simulink model "Tachometer"  (R2016b)
settings: Solver=FixedStepDiscrete  StartTime=0.0  StopTime=10  FixedStep=TimeSteps.ModelStep  RelTol=1e-3
InitFcn:
  | BusInit;
undefined symbols (not defined in the file): DiscIntNeverNeededParam, TimeSteps
settings Model: Creator=KIRTACA  LastModifiedBy=KIRTACA
settings ModelReferenceCC: UpdateModelReferenceTargets=IfOutOfDate  EnableRefExpFcnMdlSchedulingChecks=off  ModelReferenceNumInstancesAllowed=Single  ModelReferenceMinAlgLoopOccurrences=on

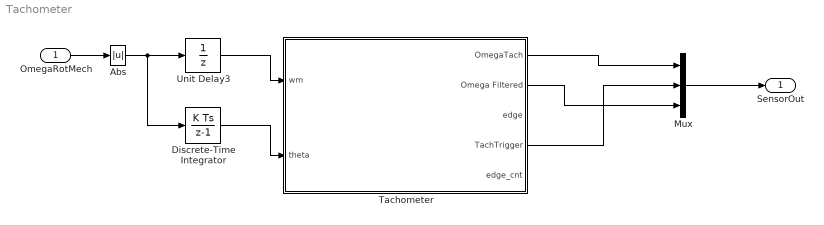
== system Tachometer ==
  OmegaRotMech : Inport  Interpolate=off
  Abs : Abs
  Discrete-Time Integrator : DiscreteIntegrator  InitialConditionSetting=State (most efficient)  SampleTime=-1  ICPrevOutput=DiscIntNeverNeededParam  ICPrevScaledInput=DiscIntNeverNeededParam
  Mux : Mux  Inputs=3
  Tachometer : Subsystem  mask(Tachometer){Clock=1e-6, p=8, tmr_bits=16, Ts=TimeSteps.ModelStep, wmax=4990*2*pi, freq_tmr=1e6, TsSlow=1/500, FirTaps=16}
      mask prompts: FirTaps "Taps"
      mask init:
      | params.Clock     = Clock;
      |         params.p         = p;
      |         params.tmr_bits  = tmr_bits;
      |         params.Ts        = Ts;
      |         params.wmax      = wmax;
      |         params.freq_tmr  = freq_tmr;
      |         params.omega_scl = 0;
      |         params.Speed_max = 0;
      |         params.FirTaps = FirTaps;
  Unit Delay3 : UnitDelay  SampleTime=-1
  SensorOut : Outport
  wires:
  Unit Delay3/1 -> Tachometer/1(wm)
  Discrete-Time Integrator/1 -> Tachometer/2("theta ")
  Abs/1 -> Discrete-Time Integrator/1, Unit Delay3/1
  Mux/1 -> SensorOut/1
  Tachometer/1(OmegaTach) -> Mux/1
  Tachometer/4(TachTrigger) -> Mux/2
  Tachometer/2(Omega Filtered) -> Mux/3
  OmegaRotMech/1 -> Abs/1

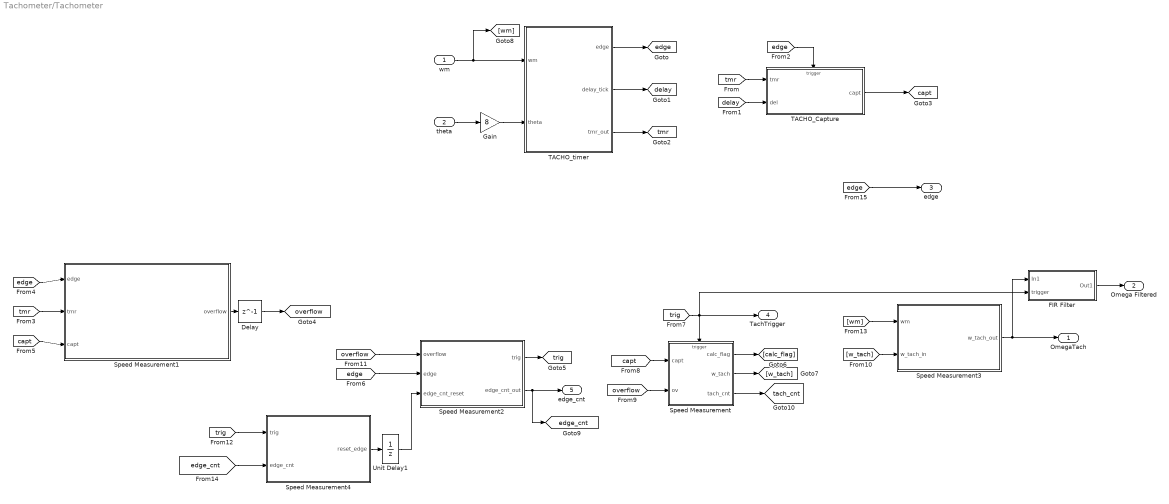
== system Tachometer/Tachometer ==
  wm : Inport
  "theta " : Inport  Port=2
  Delay : Delay  DelayLength=1  InitialCondition=0
  FIR Filter : Subsystem  TreatAsAtomicUnit=on
  Gain : Gain  Gain=8
  Speed Measurement : Subsystem  TreatAsAtomicUnit=on
  Speed Measurement1 : MATLAB Function  TreatAsAtomicUnit=on
  Speed Measurement2 : MATLAB Function  TreatAsAtomicUnit=on
  Speed Measurement3 : MATLAB Function  TreatAsAtomicUnit=on
  Speed Measurement4 : MATLAB Function  TreatAsAtomicUnit=on
  TACHO_Capture : Subsystem  TreatAsAtomicUnit=on
  TACHO_timer : MATLAB Function  TreatAsAtomicUnit=on
  Unit Delay1 : UnitDelay  SampleTime=-1
  OmegaTach : Outport
  Omega Filtered : Outport  Port=2
  edge : Outport  Port=3
  TachTrigger : Outport  Port=4
  edge_cnt : Outport  Port=5
  tag scope: capt=global, delay=global, edge=global, edge_cnt=global, overflow=global, tach_cnt=global, tmr=global, trig=global
  wires:
  Gain/1 -> TACHO_timer/2(theta)
  "theta "/1 -> Gain/1
  [overflow] -> Speed Measurement2/1(overflow)
  wm/1 -> TACHO_timer/1(wm), [wm]
  [overflow] -> Speed Measurement/2(ov)
  [capt] -> Speed Measurement/1(capt)
  [trig] -> TachTrigger/1, FIR Filter/2(trigger), Speed Measurement/Trigger
  Speed Measurement2/1(trig) -> [trig]
  [edge] -> Speed Measurement2/2(edge)
  [capt] -> Speed Measurement1/3(capt)
  [edge] -> Speed Measurement1/1(edge)
  [tmr] -> Speed Measurement1/2(tmr)
  TACHO_Capture/1(capt) -> [capt]
  [edge] -> TACHO_Capture/Trigger
  [tmr] -> TACHO_Capture/1(tmr)
  TACHO_timer/3(tmr_out) -> [tmr]
  TACHO_timer/2(delay_tick) -> [delay]
  TACHO_timer/1(edge) -> [edge]
  Speed Measurement/1(calc_flag) -> [calc_flag]
  Speed Measurement/2(w_tach) -> [w_tach]
  [delay] -> TACHO_Capture/2(del)
  [w_tach] -> Speed Measurement3/2(w_tach_in)
  Speed Measurement3/1(w_tach_out) -> OmegaTach/1, FIR Filter/1(In1)
  [wm] -> Speed Measurement3/1(wm)
  Speed Measurement2/2(edge_cnt_out) -> edge_cnt/1, [edge_cnt]
  Speed Measurement4/1(reset_edge) -> Unit Delay1/1
  [trig] -> Speed Measurement4/1(trig)
  [edge] -> edge/1
  [edge_cnt] -> Speed Measurement4/2(edge_cnt)
  Unit Delay1/1 -> Speed Measurement2/3(edge_cnt_reset)
  Speed Measurement/3(tach_cnt) -> [tach_cnt]
  Speed Measurement1/1(overflow) -> Delay/1
  Delay/1 -> [overflow]
  FIR Filter/1(Out1) -> Omega Filtered/1

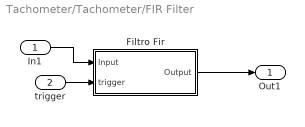
== system Tachometer/Tachometer/FIR Filter ==
  In1 : Inport
  trigger : Inport  Port=2
  Filtro Fir : Subsystem  TreatAsAtomicUnit=on
  Out1 : Outport
  wires:
  In1/1 -> Filtro Fir/1(Input)
  Filtro Fir/1(Output) -> Out1/1
  trigger/1 -> Filtro Fir/2(trigger)

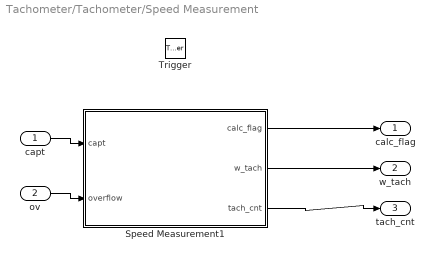
== system Tachometer/Tachometer/Speed Measurement ==
  capt : Inport
  ov : Inport  Port=2
  Trigger : TriggerPort  VariantControl=Variant
  Speed Measurement1 : MATLAB Function  TreatAsAtomicUnit=on
  calc_flag : Outport
  w_tach : Outport  Port=2
  tach_cnt : Outport  Port=3
  wires:
  Speed Measurement1/2(w_tach) -> w_tach/1
  Speed Measurement1/1(calc_flag) -> calc_flag/1
  ov/1 -> Speed Measurement1/2(overflow)
  capt/1 -> Speed Measurement1/1(capt)
  Speed Measurement1/3(tach_cnt) -> tach_cnt/1

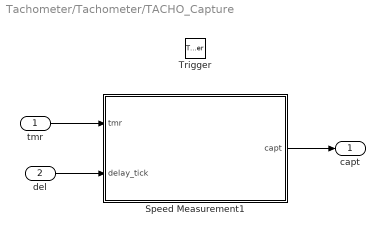
== system Tachometer/Tachometer/TACHO_Capture ==
  tmr : Inport
  del : Inport  Port=2
  Trigger : TriggerPort  VariantControl=Variant
  Speed Measurement1 : MATLAB Function  TreatAsAtomicUnit=on
  capt : Outport
  wires:
  del/1 -> Speed Measurement1/2(delay_tick)
  Speed Measurement1/1(capt) -> capt/1
  tmr/1 -> Speed Measurement1/1(tmr)

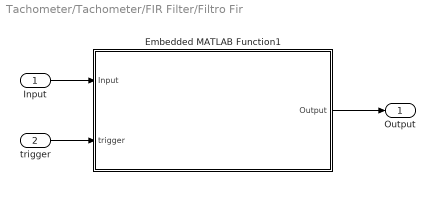
== system Tachometer/Tachometer/FIR Filter/Filtro Fir ==
  Input : Inport
  trigger : Inport  Port=2
  Embedded MATLAB Function1 : MATLAB Function  TreatAsAtomicUnit=on
  Output : Outport
  wires:
  Input/1 -> Embedded MATLAB Function1/1(Input)
  Embedded MATLAB Function1/1(Output) -> Output/1
  trigger/1 -> Embedded MATLAB Function1/2(trigger)

== matlab function Tachometer/FIR Filter/Filtro Fir/Embedded MATLAB Function1 ==
  data: params parameter; Output output; Input input; trigger input
function Output  = FiltroFir(params, Input,trigger)
%#eml
persistent Buffer;
persistent FilterIndex;
persistent Output_holder;

if isempty(Buffer)
    Buffer = zeros(32,1);
end

if isempty(FilterIndex)
    FilterIndex = 1;
end
    
if isempty(Output_holder)
    Output_holder = 0;
end

Taps = params.FirTaps;


if (trigger == 1)
    if(FilterIndex > Taps)
        FilterIndex = 1;
    end

    Buffer(FilterIndex,1) = Input;

    FilterIndex = FilterIndex+1;

    Output_holder = 0;
    for i= 1:Taps
    Output_holder = Output_holder+ Buffer(i,1)/Taps;
    end
end

Output = Output_holder;

== matlab function Tachometer/Speed Measurement/Speed Measurement1 ==
  data: params parameter; calc_flag output; capt input; overflow input; w_tach output; tach_cnt output
function [calc_flag, w_tach, tach_cnt]   = speed_meas(params,capt,overflow)
persistent capt_state w_tach_state
%#codegen
if isempty(capt_state)
    capt_state = 0;
    w_tach_state = 0;
end

tmr_bits = params.tmr_bits;
freq_tmr = params.freq_tmr;
p        = params.p;

omega_scl = freq_tmr/(2*p)*2*pi;
Speed_max = 10000/2*2*p/60*(2*pi); % [rad/s]

tach_cnt_min = round(omega_scl/Speed_max); % for fixed point is directly omega_scl

% update the difference
if (overflow == 0)
    tach_cnt = capt - capt_state;
else
    tach_cnt = 2^tmr_bits - capt_state + capt;
end

if tach_cnt<0
    tach_cnt = tach_cnt + 2^tmr_bits;
end

w_tmp = 0;
% min tach count logic
if tach_cnt > tach_cnt_min;
    calc_flag = 1;       
    w_tmp = omega_scl/tach_cnt;  %[rad/s]    
else
    calc_flag = -1;
    % update min tach failure counter
    % ....    
end

% overflow handler
if overflow > 1    
    calc_flag = 0; 
end
    
%update the mem value
capt_state = capt;

switch calc_flag
    case -1
        w_tach = w_tach_state;
    case 0
        w_tach = 0;
        
    otherwise
        w_tach = w_tmp;
end

w_tach_state = w_tach;

== matlab function Tachometer/Speed Measurement1 ==
  data: edge input; tmr input; capt input; overflow output
function overflow = overflow_mgr(edge,tmr,capt)
persistent overflow_state
%#codegen

if isempty(overflow_state)
    overflow_state = 3;
end


if edge == 1
    if (overflow_state == 3)
        % discard first edge
         overflow = 2;
    else
        overflow = 0;
    end
else
    switch overflow_state
        case 0
            if (capt >= tmr)
                overflow = 1;
            else
                overflow = overflow_state;
            end
        case 1
            if (capt <= tmr)
                overflow = 2;
            else
                overflow = overflow_state;
            end

        otherwise
            overflow = overflow_state;
    end
end
overflow_state = overflow;

== matlab function Tachometer/Speed Measurement2 ==
  data: overflow input; edge input; trig output; edge_cnt_reset input; edge_cnt_out output
function [trig, edge_cnt_out]   = speed_meas_trig(overflow, edge, edge_cnt_reset)
persistent edge_cnt
%#codegen
if isempty(edge_cnt)
    edge_cnt = 0;
end

if (edge_cnt_reset == 1)
    edge_cnt = 0;
end

if (edge == 1) %|| (overflow>1)
    trig = 1;   
else
    trig = 0;    
end

if (edge == 1)
    edge_cnt = edge_cnt + 1; 
end

edge_cnt_out = edge_cnt;

== matlab function Tachometer/Speed Measurement3 ==
  data: params parameter; wm input; w_tach_in input; w_tach_out output
function w_tach_out    = high_speed_simplified(params,wm, w_tach_in)
%#codegen

wm = abs(wm);

% threshold speed for correct tacho model simulation result
if ((wm / (2*pi)) < (0.9 / params.Ts / (4 * params.p)))
    w_tach_out = w_tach_in;
else
    w_tach_out = wm;
end

== matlab function Tachometer/Speed Measurement4 ==
  data: params parameter; trig input; reset_edge output double; edge_cnt input
function reset_edge    = edge_cnt_reset(params, trig, edge_cnt)
persistent cnt
%#codegen

Ts =  params.Ts;
reset_edge = 0;

if isempty(cnt)
    cnt = 0;
end

if (trig == 1)
    cnt = 0;
else
    cnt = cnt + 1;
end

if (cnt > (0.5/Ts))  % no event in 0.5s
    if (edge_cnt > 10) % we are in close loop for sure
        reset_edge = 1;
    else
        reset_edge = 0;
    end
else
    reset_edge = 0;
end

== matlab function Tachometer/TACHO_Capture/Speed Measurement1 ==
  data: tmr input; capt output; delay_tick input
function capt = capt_meas(tmr, delay_tick)
%#codegen

% update capture value
capt = tmr - delay_tick;

== matlab function Tachometer/TACHO_timer ==
  data: params parameter; edge output; delay_tick output; wm input; theta input; tmr_out output
function [edge, delay_tick, tmr_out] = timer(params,wm, theta)
persistent state tmr
%#codegen
clock = params.Clock;
p = params.p;
Ts =  params.Ts;
tmr_bits = params.tmr_bits;
wmax =  params.wmax;
if isempty(state)
    state = 0;
    tmr = 0;
end
    
if (2*p*wm)>wmax
    wm = wmax/(2*p);
end


%wm is in [rad/s]
tacho_wave = sin(theta);
tmr = tmr + round(Ts/clock);
tmr = rem(tmr,2^tmr_bits);

state_old = state;
%state = state_old;
% zero crossing detection
if state == 0
    if tacho_wave >= 0
        state = 1;
    end
else
    if tacho_wave < 0
        state = 0;
    end
end
% wm = wtach;
if state_old ~= state
    % update edge flag
    edge = 1;    
    % correction term
    if wm == 0
        delay_tick = 0;
    else
        delay = asin(abs(tacho_wave)); % rad
        delay_t = delay/(p*wm); % s
        delay_tick = round(delay_t/clock);
    end
else
    edge = 0;
    delay_tick = 0;
end

tmr_out = tmr;
